simulink model "P2"  (R2020b)
settings: Solver=VariableStepAuto  StartTime=0.0  StopTime=10.0  RelTol=1e-3
settings Model: Creator=ASUS  LastModifiedBy=ASUS

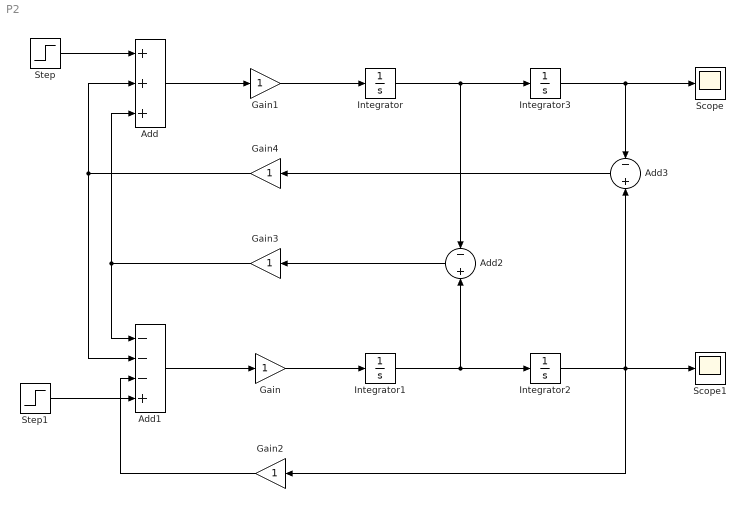
== system P2 ==
  Add : Sum  Inputs=+++
  Add1 : Sum  Inputs=---+
  Add2 : Sum  Inputs=-+
  Add3 : Sum  Inputs=-+
  Gain{,1..4} (5 alike) : Gain
  Integrator{,1..3} (4 alike) : Integrator
  Scope : Scope
  Scope1 : Scope
  Step : Step  After=450  SampleTime=0
  Step1 : Step  After=150  SampleTime=0
  wires:
  Add/1 -> Gain1/1
  Gain1/1 -> Integrator/1
  Add1/1 -> Gain/1
  Gain/1 -> Integrator1/1
  Gain2/1 -> Add1/3
  Add2/1 -> Gain3/1
  Add3/1 -> Gain4/1
  Integrator/1 -> Add2/1, Integrator3/1
  Integrator3/1 -> Add3/1, Scope/1
  Integrator1/1 -> Add2/2, Integrator2/1
  Integrator2/1 -> Gain2/1, Scope1/1, Add3/2
  Gain4/1 -> Add1/2, Add/2
  Gain3/1 -> Add1/1, Add/3
  Step/1 -> Add/1
  Step1/1 -> Add1/4
